simulink model "ModeAdjust"  (R2018b)
settings: Solver=FixedStepDiscrete  StartTime=0.0  StopTime=inf  FixedStep=0.01  RelTol=1e-3
undefined symbols (not defined in the file or in its folder): IfKeSMSbSeatMovBkRclnEnable_Val, IfKeSMSbSeatMovFrwdBkwdEnable_Val, IfKeSMSbSeatMovFtrstEnable_Val, IfKeSMSbSeatMovHdrstFrwdBkwdEnable_Val, IfKeSMSbSeatMovHdUpwdDnwdEnable_Val, IfKeSMSbSeatMovLgrstEnable_Val, IfKeSMSbSeatMovLtwdRtwdEnable_Val, IfVeSMSeStNumConfig, KeSMSbArmscreenMovEnable_Val, KeSMSbSeatMovLgrstExpdEnable_Val, KeSMSuFirstRwStBackPosDelta_Val, KeSMSuFirstRwStBackPosTolr_Val, KeSMSuFirstRwStCushFrntPosDelta_Val, KeSMSuFirstRwStCushFrntPosTolr_Val, KeSMSuFirstRwStCushRePosDelta_Val, KeSMSuFirstRwStCushRePosTolr_Val, KeSMSuFirstRwStFootrestPosDelta_Val, KeSMSuFirstRwStFootrestPosTolr_Val, KeSMSuFirstRwStFwdBkwdPosDelta_Val, KeSMSuFirstRwStFwdBkwdPosTolr_Val, KeSMSuMdMotFinshdTm_Val, KeSMSuMdRetryTm1_Val, KeSMSuModeReqDurgTm_Val, KeSMSuSecRwStArmTochPosDelta_Val, KeSMSuSecRwStArmTochPosTolr_Val, KeSMSuSecRwStBackPosDelta_Val, KeSMSuSecRwStBackPosTolr_Val, KeSMSuSecRwStFtrstUpwdDnwdPosDelta_Val, KeSMSuSecRwStFtrstUpwdDnwdPosTolr_Val, KeSMSuSecRwStFwdBkwdPosDelta_Val, KeSMSuSecRwStFwdBkwdPosTolr_Val, KeSMSuSecRwStHeadrestFwdBkwdPosDelta_Val, KeSMSuSecRwStHeadrestFwdBkwdPosTolr_Val, KeSMSuSecRwStHeadrestUpwdDwnwdPosDelta_Val, KeSMSuSecRwStHeadrestUpwdDwnwdPosTolr_Val, KeSMSuSecRwStLegrestInOutPosDelta_Val, KeSMSuSecRwStLegrestInOutPosTolr_Val, KeSMSuSecRwStLegrestUpwdDwnwdPosDelta_Val, KeSMSuSecRwStLegrestUpwdDwnwdPosTolr_Val, KeSMSuSecRwStLwdRwdPosDelta_Val, KeSMSuSecRwStLwdRwdPosTolr_Val, KeSMSuSecRwStVIPFtrstRefAngle_Val, KeSMSuThirdRwStFwdBkwdPosDelta_Val, KeSMSuThirdRwStFwdBkwdPosTolr_Val, KeSMSuThrdRwCushFoldPosDelta_Val, KeSMSuThrdRwCushFoldPosTolr_Val, KeSMSuThrdRwStBackPosDelta_Val, KeSMSuThrdRwStBackPosTolr_Val, KeSMSw4SLegrstCloseMdSecRwLtStFtrstUpwdDnwdPos_Val, KeSMSw4SLegrstCloseMdSecRwLtStFtrstUpwdDnwdPosMax_Val, KeSMSw4SLegrstCloseMdSecRwLtStFtrstUpwdDnwdPosMin_Val, KeSMSw4SLegrstCloseMdSecRwLtStLgrstOtwdInwdPos_Val, KeSMSw4SLegrstCloseMdSecRwLtStLgrstOtwdInwdPosMax_Val, KeSMSw4SLegrstCloseMdSecRwLtStLgrstOtwdInwdPosMin_Val, KeSMSw4SLegrstCloseMdSecRwLtStLgrstUpwdDnwdPos_Val, KeSMSw4SLegrstCloseMdSecRwLtStLgrstUpwdDnwdPosMax_Val, KeSMSw4SLegrstCloseMdSecRwLtStLgrstUpwdDnwdPosMin_Val, KeSMSw4SLegrstCloseMdSecRwRtStFtrstUpwdDnwdPos_Val, KeSMSw4SLegrstCloseMdSecRwRtStFtrstUpwdDnwdPosMax_Val, KeSMSw4SLegrstCloseMdSecRwRtStFtrstUpwdDnwdPosMin_Val ... (+1138)
libraries: Lib x401
(part 35 of 35)

== stateflow chart ModeAdjust/ModeAdjustRunnable_sys/ModeAdjust/RecvyR4s/Chart ==
  (default) -> (junction 3) : {failflg=0;}
  (junction 3) -> (junction 5) [order 1] : [!R2Lt_ini]
  (junction 5) -> (junction 9) [order 1] : [R2Lt_done]
  (junction 3) -> (junction 13) [order 2] : {R2Lt_En=false;}
  (junction 5) -> (junction 7) [order 2] : {R2Lt_En=true;}
  (junction 9) -> (junction 11) : {R2Lt_En=false;}
  (junction 7) -> (junction 13)
  (junction 11) -> (junction 7)
  (junction 13) -> (junction 237)
  (junction 237) -> (junction 244) [order 1] : [!HdUp_ini]
  (junction 244) -> (junction 234) [order 1] : [HdUp_Done]
  (junction 237) -> (junction 235) [order 2] : {HdUp_En =false;}
  (junction 244) -> (junction 246) [order 2] : {HdUp_En = true;}
  (junction 234) -> (junction 236) : {HdUp_En =false;}
  (junction 246) -> (junction 235)
  (junction 236) -> (junction 246)
  (junction 235) -> (junction 62)
  (junction 62) -> (junction 105) [order 1] : [!Step1_ini]
  (junction 105) -> (junction 107) [order 1] : [Step1done]
  (junction 62) -> (junction 68) [order 2] : {
      | StepEn_LgrstStep1=false;
      | }
  (junction 105) -> (junction 82) [order 2] : {StepEn_LgrstStep1=true;}
  (junction 107) -> (junction 109) : {StepEn_LgrstStep1=false;}
  (junction 82) -> (junction 68)
  (junction 109) -> (junction 82)
  (junction 68) -> (junction 143)
  (junction 143) -> (junction 142) [order 1] : [!Step2_ini]
  (junction 142) -> (junction 157) [order 1] : [downpos<=closedownpos2&&Ftpos>=FtposDelta]
  (junction 157) -> (junction 224) [order 1] : [Step1done&&Step3done]
  (junction 143) -> (junction 89) [order 2] : {
      | StepEn_LgrstStep2=false;
      | }
  (junction 142) -> (junction 154) [order 2]
  (junction 157) -> (junction 159) [order 2] : {
      | StepEn_LgrstStep2=false;
      | }
  (junction 224) -> (junction 228) : {failflg=1;}
  (junction 154) -> (junction 148) [order 1] : [downpos<closedownpos1&&Otpos>closeOtpos1]
  (junction 154) -> (junction 87) [order 2]
  (junction 148) -> (junction 150) : {StepEn_LgrstStep2 = false;}
  (junction 87) -> (junction 94) [order 1] : [Step2done]
  (junction 87) -> (junction 91) [order 2] : {
      | StepEn_LgrstStep2=true;
      | }
  (junction 94) -> (junction 96) : {
      | StepEn_LgrstStep2=false;
      | }
  (junction 91) -> (junction 89)
  (junction 96) -> (junction 91)
  (junction 150) -> (junction 96)
  (junction 159) -> (junction 150)
  (junction 228) -> (junction 159)
  (junction 89) -> (junction 101)
  (junction 101) -> (junction 113) [order 1] : [!Step3_ini]
  (junction 113) -> (junction 115) [order 1] : [Step3done||!Step1done]
  (junction 101) -> (junction 118) [order 2] : {
      | StepEn_LgrstStep3=false;
      | }
  (junction 113) -> (junction 258) [order 2]
  (junction 115) -> (junction 122) : {
      | StepEn_LgrstStep3=false;
      | }
  (junction 258) -> (junction 260) [order 1] : [downpos>closedownpos2]
  (junction 260) -> (junction 274) [order 1] : [Step2done]
  (junction 258) -> (junction 116) [order 2] : {
      | StepEn_LgrstStep3=true;
      | }
  (junction 260) -> (junction 262) [order 2] : {StepEn_LgrstStep3 = false;}
  (junction 274) -> (junction 276) : {
      | StepEn_LgrstStep3=true;
      | }
  (junction 116) -> (junction 118)
  (junction 262) -> (junction 116)
  (junction 276) -> (junction 262)
  (junction 122) -> (junction 276)
  (junction 118) -> (junction 182)
  (junction 182) -> (junction 178) [order 1] : [(Step1done&&Step2done&&Step3done)||failflg==1]
  (junction 178) -> (junction 252) [order 1] : [!HFwd_ini]
  (junction 252) -> (junction 173) [order 1] : [HdFwd_Done]
  (junction 182) -> (junction 181) [order 2]
  (junction 178) -> (junction 174) [order 2] : {HdFwd_En =false;}
  (junction 252) -> (junction 254) [order 2] : {HdFwd_En =true;}
  (junction 173) -> (junction 175) : {HdFwd_En =false;}
  (junction 254) -> (junction 174)
  (junction 175) -> (junction 254)
  (junction 174) -> (junction 176)
  (junction 176) -> (junction 181)
  (junction 181) -> (junction 165)
  data: R2Lt_ini input boolean; R2Lt_done input boolean; R2Lt_En output boolean; downpos input uint16; Otpos input uint16; Ftpos input uint16; closedownpos1 input uint16; closedownpos2 input uint16; closeOtpos1 input uint16; Step1done input boolean; Step2done input boolean; Step3done input boolean; Step1_ini input boolean; Step2_ini input boolean; Step3_ini input boolean; StepEn_LgrstStep1 output boolean; StepEn_LgrstStep2 output boolean; StepEn_LgrstStep3 output boolean; FtposDelta input uint16; HdFwd_Done input boolean; HdUp_Done input boolean; HdUp_En output boolean; HdFwd_En output boolean; OtposDelta input uint16; failflg output boolean; HdUp_ini input boolean; HFwd_ini input boolean

== stateflow chart ModeAdjust/ModeAdjustRunnable_sys/ModeAdjust/RecvyR4s/Chart1 ==
  (default) -> (junction 1)
  (junction 1) -> (junction 3) [order 1] : [Left_Done]
  (junction 1) -> (junction 7) [order 2] : {
      | IfVeSMSuSecRwLtStRclCmdSrv_Val_write=IfVeSMSuSecRwLtStRclCmdSrv_Val_writeRaw;
      | Md_L_DoneOk=false;
      | Md_L_DoneFailed=false;
      | }
  (junction 3) -> (junction 5) : {
      | IfVeSMSuSecRwLtStRclCmdSrv_Val_write=false;
      | Md_L_DoneOk=Md_L_DoneOkRaw;
      | Md_L_DoneFailed=Md_L_DoneFailedRaw;
      | }
  (junction 5) -> (junction 7)
  (junction 7) -> (junction 10)
  data: Left_Done input boolean; IfVeSMSuSecRwLtStRclCmdSrv_Val_write output boolean; IfVeSMSuSecRwLtStRclCmdSrv_Val_writeRaw input; Md_L_DoneOkRaw input; Md_L_DoneFailedRaw input; Md_L_DoneOk output boolean; Md_L_DoneFailed output boolean

== stateflow chart ModeAdjust/ModeAdjustRunnable_sys/ModeAdjust/INTMR/Chart ==
  (default) -> (junction 10)
  (junction 10) -> (junction 58) [order 1] : [!L_R2_ini]
  (junction 58) -> (junction 25) [order 1] : [L_R2_done]
  (junction 10) -> (junction 26) [order 2] : {L_R2_en=false;}
  (junction 58) -> (junction 35) [order 2] : {L_R2_en=true;}
  (junction 25) -> (junction 18) : {
      | L_R2_en=false;
      | }
  (junction 35) -> (junction 26)
  (junction 18) -> (junction 35)
  (junction 26) -> (junction 129)
  (junction 129) -> (junction 133) [order 1] : [!R_R2_ini]
  (junction 133) -> (junction 128) [order 1] : [R_R2_done]
  (junction 129) -> (junction 131) [order 2] : {R_R2_en=false;}
  (junction 133) -> (junction 127) [order 2] : {R_R2_en=true;}
  (junction 128) -> (junction 125) : {
      | R_R2_en=false;
      | }
  (junction 127) -> (junction 131)
  (junction 125) -> (junction 127)
  (junction 131) -> (junction 134)
  data: L_R2_ini input boolean; L_R2_done input boolean; R_R2_en output boolean; L_R2_en output boolean; R_R2_ini input boolean; R_R2_done input boolean

== stateflow chart ModeAdjust/ModeAdjustRunnable_sys/ModeAdjust/INTMR/Chart1 ==
  (default) -> (junction 1)
  (junction 1) -> (junction 3) [order 1] : [StepAlldone]
  (junction 1) -> (junction 7) [order 2] : {
      | IfVeSMSbSecRwRtStRclCmdSrv_Val_write=IfVeSMSbSecRwRtStRclCmdSrv_Val_writeRaw;
      | IfVeSMSuSecRwLtStRclCmdSrv_Val_write=IfVeSMSuSecRwLtStRclCmdSrv_Val_writeRaw;
      | isINTMDoneOk=false;
      | isINTMDoneFailed=false;
      | }
  (junction 3) -> (junction 5) : {
      | IfVeSMSbSecRwRtStRclCmdSrv_Val_write=false;
      | IfVeSMSuSecRwLtStRclCmdSrv_Val_write=false;
      | isINTMDoneOk=isINTMDoneOkRaw;
      | isINTMDoneFailed=isINTMDoneFailedRaw;
      | }
  (junction 5) -> (junction 7)
  (junction 7) -> (junction 10)
  data: StepAlldone input boolean; IfVeSMSbSecRwRtStRclCmdSrv_Val_write output boolean; IfVeSMSuSecRwLtStRclCmdSrv_Val_write output boolean; isINTMDoneOk output boolean; isINTMDoneFailed output boolean; IfVeSMSbSecRwRtStRclCmdSrv_Val_writeRaw input; IfVeSMSuSecRwLtStRclCmdSrv_Val_writeRaw input; isINTMDoneFailedRaw input; isINTMDoneOkRaw input

== stateflow chart ModeAdjust/ModeAdjustRunnable_sys/ModeAdjust/LgrstCloseL/Chart ==
  (default) -> (junction 62) : {failflg=0;}
  (junction 62) -> (junction 105) [order 1] : [!Step1_ini]
  (junction 105) -> (junction 107) [order 1] : [Step1done]
  (junction 62) -> (junction 68) [order 2] : {
      | StepEn_LgrstStep1=false;
      | }
  (junction 105) -> (junction 82) [order 2] : {StepEn_LgrstStep1=true;}
  (junction 107) -> (junction 109) : {StepEn_LgrstStep1=false;}
  (junction 82) -> (junction 68)
  (junction 109) -> (junction 82)
  (junction 68) -> (junction 143)
  (junction 143) -> (junction 142) [order 1] : [!Step2_ini]
  (junction 142) -> (junction 157) [order 1] : [downpos<=closedownpos2&&Ftpos>=FtposDelta]
  (junction 157) -> (junction 224) [order 1] : [Step1done&&Step3done]
  (junction 143) -> (junction 89) [order 2] : {
      | StepEn_LgrstStep2=false;
      | }
  (junction 142) -> (junction 154) [order 2]
  (junction 157) -> (junction 159) [order 2] : {
      | StepEn_LgrstStep2=false;
      | }
  (junction 224) -> (junction 228) : {failflg=1;}
  (junction 154) -> (junction 148) [order 1] : [downpos<closedownpos1&&Otpos>closeOtpos1]
  (junction 154) -> (junction 87) [order 2]
  (junction 148) -> (junction 150) : {StepEn_LgrstStep2 = false;}
  (junction 87) -> (junction 94) [order 1] : [Step2done]
  (junction 87) -> (junction 91) [order 2] : {
      | StepEn_LgrstStep2=true;
      | }
  (junction 94) -> (junction 96) : {
      | StepEn_LgrstStep2=false;
      | }
  (junction 91) -> (junction 89)
  (junction 96) -> (junction 91)
  (junction 150) -> (junction 96)
  (junction 159) -> (junction 150)
  (junction 228) -> (junction 159)
  (junction 89) -> (junction 101)
  (junction 101) -> (junction 113) [order 1] : [!Step3_ini]
  (junction 113) -> (junction 115) [order 1] : [Step3done||!Step1done]
  (junction 101) -> (junction 118) [order 2] : {
      | StepEn_LgrstStep3=false;
      | }
  (junction 113) -> (junction 215) [order 2]
  (junction 115) -> (junction 122) : {
      | StepEn_LgrstStep3=false;
      | }
  (junction 215) -> (junction 217) [order 1] : [downpos>closedownpos2]
  (junction 217) -> (junction 259) [order 1] : [Step2done]
  (junction 215) -> (junction 116) [order 2] : {
      | StepEn_LgrstStep3=true;
      | }
  (junction 217) -> (junction 219) [order 2] : {
      | StepEn_LgrstStep3=false;
      | }
  (junction 259) -> (junction 261) : {
      | StepEn_LgrstStep3=true;
      | }
  (junction 116) -> (junction 118)
  (junction 219) -> (junction 116)
  (junction 261) -> (junction 219)
  (junction 122) -> (junction 261)
  (junction 118) -> (junction 182)
  data: downpos input uint16; Otpos input uint16; Ftpos input uint16; closedownpos1 input uint16; closedownpos2 input uint16; closeOtpos1 input uint16; Step1done input boolean; Step2done input boolean; Step3done input boolean; Step1_ini input boolean; Step2_ini input boolean; Step3_ini input boolean; StepEn_LgrstStep1 output boolean; StepEn_LgrstStep2 output boolean; StepEn_LgrstStep3 output boolean; FtposDelta input uint16; OtposDelta input uint16; failflg output boolean

== stateflow chart ModeAdjust/ModeAdjustRunnable_sys/ModeAdjust/LgrstCloseL/Chart1 ==
  (default) -> (junction 1)
  (junction 1) -> (junction 3) [order 1] : [Left_Done]
  (junction 1) -> (junction 7) [order 2] : {
      | IfVeSMSuSecRwLtStRclCmdSrv_Val_write=IfVeSMSuSecRwLtStRclCmdSrv_Val_writeRaw;
      | Md_L_DoneOk=false;
      | Md_L_DoneFailed=false;
      | }
  (junction 3) -> (junction 5) : {
      | IfVeSMSuSecRwLtStRclCmdSrv_Val_write=false;
      | Md_L_DoneOk=Md_L_DoneOkRaw;
      | Md_L_DoneFailed=Md_L_DoneFailedRaw;
      | }
  (junction 5) -> (junction 7)
  (junction 7) -> (junction 10)
  data: Left_Done input boolean; IfVeSMSuSecRwLtStRclCmdSrv_Val_write output boolean; IfVeSMSuSecRwLtStRclCmdSrv_Val_writeRaw input; Md_L_DoneOkRaw input; Md_L_DoneFailedRaw input; Md_L_DoneOk output boolean; Md_L_DoneFailed output boolean

== stateflow chart ModeAdjust/ModeAdjustRunnable_sys/ModeAdjust/LgrstOpenL/Chart ==
  (default) -> (junction 182) : {failflg =0;}
  (junction 182) -> (junction 62)
  (junction 62) -> (junction 76) [order 1] : [!Step1_ini]
  (junction 76) -> (junction 64) [order 1] : [pos<openpos1]
  (junction 64) -> (junction 74) [order 1] : [Step1done]
  (junction 62) -> (junction 68) [order 2] : {
      | StepEn_LgrstStep1=false;
      | }
  (junction 76) -> (junction 105) [order 2]
  (junction 64) -> (junction 66) [order 2] : {
      | StepEn_LgrstStep1=true;
      | StepEn_LgrstStep2=false;
      | StepEn_LgrstStep3=false;
      | }
  (junction 74) -> (junction 102) : {
      | StepEn_LgrstStep1=false;
      | StepEn_LgrstStep2=false;
      | StepEn_LgrstStep3=false;
      | failflg =1;
      | }
  (junction 105) -> (junction 107) [order 1] : [!Step2done||Step1done]
  (junction 105) -> (junction 82) [order 2] : {StepEn_LgrstStep1=true;}
  (junction 107) -> (junction 109) : {StepEn_LgrstStep1=false;}
  (junction 82) -> (junction 68)
  (junction 109) -> (junction 82)
  (junction 102) -> (junction 66)
  (junction 68) -> (junction 85)
  (junction 66) -> (junction 99)
  (junction 85) -> (junction 87) [order 1] : [!Step2_ini]
  (junction 87) -> (junction 94) [order 1] : [Step2done]
  (junction 85) -> (junction 89) [order 2] : {
      | StepEn_LgrstStep2=false;
      | }
  (junction 87) -> (junction 91) [order 2] : {
      | StepEn_LgrstStep2=true;
      | }
  (junction 94) -> (junction 96) : {
      | StepEn_LgrstStep2=false;
      | }
  (junction 91) -> (junction 89)
  (junction 96) -> (junction 91)
  (junction 89) -> (junction 101)
  (junction 101) -> (junction 113) [order 1] : [!Step3_ini]
  (junction 113) -> (junction 115) [order 1] : [(!Step2done)||Step3done]
  (junction 101) -> (junction 118) [order 2] : {
      | StepEn_LgrstStep3=false;
      | }
  (junction 113) -> (junction 116) [order 2] : {
      | StepEn_LgrstStep3=true;
      | }
  (junction 115) -> (junction 122) : {
      | StepEn_LgrstStep3=false;
      | }
  (junction 116) -> (junction 118)
  (junction 122) -> (junction 116)
  (junction 99) -> (junction 122)
  (junction 118) -> (junction 166)
  data: pos input uint16; openpos1 input uint16; Step1done input boolean; Step2done input boolean; Step3done input boolean; Step1_ini input boolean; Step2_ini input boolean; Step3_ini input boolean; StepEn_LgrstStep1 output boolean; StepEn_LgrstStep2 output boolean; StepEn_LgrstStep3 output boolean; failflg output boolean

== stateflow chart ModeAdjust/ModeAdjustRunnable_sys/ModeAdjust/LgrstOpenL/Chart1 ==
  (default) -> (junction 1)
  (junction 1) -> (junction 3) [order 1] : [Left_Done]
  (junction 1) -> (junction 7) [order 2] : {
      | IfVeSMSuSecRwLtStRclCmdSrv_Val_write=IfVeSMSuSecRwLtStRclCmdSrv_Val_writeRaw;
      | Md_L_DoneOk=false;
      | Md_L_DoneFailed=false;
      | }
  (junction 3) -> (junction 5) : {
      | IfVeSMSuSecRwLtStRclCmdSrv_Val_write=false;
      | Md_L_DoneOk=Md_L_DoneOkRaw;
      | Md_L_DoneFailed=Md_L_DoneFailedRaw;
      | }
  (junction 5) -> (junction 7)
  (junction 7) -> (junction 10)
  data: Left_Done input boolean; IfVeSMSuSecRwLtStRclCmdSrv_Val_write output boolean; IfVeSMSuSecRwLtStRclCmdSrv_Val_writeRaw input; Md_L_DoneOkRaw input; Md_L_DoneFailedRaw input; Md_L_DoneOk output boolean; Md_L_DoneFailed output boolean

== stateflow chart ModeAdjust/ModeAdjustRunnable_sys/ModeAdjust/LgrstOpenR/Chart ==
  (default) -> (junction 182) : {failflg =0;}
  (junction 182) -> (junction 62)
  (junction 62) -> (junction 76) [order 1] : [!Step1_ini]
  (junction 76) -> (junction 64) [order 1] : [pos<openpos1]
  (junction 64) -> (junction 74) [order 1] : [Step1done]
  (junction 62) -> (junction 68) [order 2] : {
      | StepEn_LgrstStep1=false;
      | }
  (junction 76) -> (junction 105) [order 2]
  (junction 64) -> (junction 66) [order 2] : {
      | StepEn_LgrstStep1=true;
      | StepEn_LgrstStep2=false;
      | StepEn_LgrstStep3=false;
      | }
  (junction 74) -> (junction 102) : {
      | StepEn_LgrstStep1=false;
      | StepEn_LgrstStep2=false;
      | StepEn_LgrstStep3=false;
      | failflg =1;
      | }
  (junction 105) -> (junction 107) [order 1] : [!Step2done||Step1done]
  (junction 105) -> (junction 82) [order 2] : {StepEn_LgrstStep1=true;}
  (junction 107) -> (junction 109) : {StepEn_LgrstStep1=false;}
  (junction 82) -> (junction 68)
  (junction 109) -> (junction 82)
  (junction 102) -> (junction 66)
  (junction 68) -> (junction 85)
  (junction 66) -> (junction 99)
  (junction 85) -> (junction 87) [order 1] : [!Step2_ini]
  (junction 87) -> (junction 94) [order 1] : [Step2done]
  (junction 85) -> (junction 89) [order 2] : {
      | StepEn_LgrstStep2=false;
      | }
  (junction 87) -> (junction 91) [order 2] : {
      | StepEn_LgrstStep2=true;
      | }
  (junction 94) -> (junction 96) : {
      | StepEn_LgrstStep2=false;
      | }
  (junction 91) -> (junction 89)
  (junction 96) -> (junction 91)
  (junction 89) -> (junction 101)
  (junction 101) -> (junction 113) [order 1] : [!Step3_ini]
  (junction 113) -> (junction 115) [order 1] : [(!Step2done)||Step3done]
  (junction 101) -> (junction 118) [order 2] : {
      | StepEn_LgrstStep3=false;
      | }
  (junction 113) -> (junction 116) [order 2] : {
      | StepEn_LgrstStep3=true;
      | }
  (junction 115) -> (junction 122) : {
      | StepEn_LgrstStep3=false;
      | }
  (junction 116) -> (junction 118)
  (junction 122) -> (junction 116)
  (junction 99) -> (junction 122)
  (junction 118) -> (junction 166)
  data: pos input uint16; openpos1 input uint16; Step1done input boolean; Step2done input boolean; Step3done input boolean; Step1_ini input boolean; Step2_ini input boolean; Step3_ini input boolean; StepEn_LgrstStep1 output boolean; StepEn_LgrstStep2 output boolean; StepEn_LgrstStep3 output boolean; failflg output boolean

== stateflow chart ModeAdjust/ModeAdjustRunnable_sys/ModeAdjust/LgrstOpenR/Chart1 ==
  (default) -> (junction 1)
  (junction 1) -> (junction 3) [order 1] : [Left_Done]
  (junction 1) -> (junction 7) [order 2] : {
      | IfVeSMSuSecRwLtStRclCmdSrv_Val_write=IfVeSMSuSecRwLtStRclCmdSrv_Val_writeRaw;
      | Md_L_DoneOk=false;
      | Md_L_DoneFailed=false;
      | }
  (junction 3) -> (junction 5) : {
      | IfVeSMSuSecRwLtStRclCmdSrv_Val_write=false;
      | Md_L_DoneOk=Md_L_DoneOkRaw;
      | Md_L_DoneFailed=Md_L_DoneFailedRaw;
      | }
  (junction 5) -> (junction 7)
  (junction 7) -> (junction 10)
  data: Left_Done input boolean; IfVeSMSuSecRwLtStRclCmdSrv_Val_write output boolean; IfVeSMSuSecRwLtStRclCmdSrv_Val_writeRaw input; Md_L_DoneOkRaw input; Md_L_DoneFailedRaw input; Md_L_DoneOk output boolean; Md_L_DoneFailed output boolean

== stateflow chart ModeAdjust/ModeAdjustRunnable_sys/ModeAdjust/LgrstCloseR/Chart ==
  (default) -> (junction 62) : {failflg=0;}
  (junction 62) -> (junction 105) [order 1] : [!Step1_ini]
  (junction 105) -> (junction 107) [order 1] : [Step1done]
  (junction 62) -> (junction 68) [order 2] : {
      | StepEn_LgrstStep1=false;
      | }
  (junction 105) -> (junction 82) [order 2] : {StepEn_LgrstStep1=true;}
  (junction 107) -> (junction 109) : {StepEn_LgrstStep1=false;}
  (junction 82) -> (junction 68)
  (junction 109) -> (junction 82)
  (junction 68) -> (junction 143)
  (junction 143) -> (junction 142) [order 1] : [!Step2_ini]
  (junction 142) -> (junction 157) [order 1] : [downpos<=closedownpos2&&Ftpos>=FtposDelta]
  (junction 157) -> (junction 224) [order 1] : [Step1done&&Step3done]
  (junction 143) -> (junction 89) [order 2] : {
      | StepEn_LgrstStep2=false;
      | }
  (junction 142) -> (junction 154) [order 2]
  (junction 157) -> (junction 159) [order 2] : {
      | StepEn_LgrstStep2=false;
      | }
  (junction 224) -> (junction 228) : {failflg=1;}
  (junction 154) -> (junction 148) [order 1] : [downpos<closedownpos1&&Otpos>closeOtpos1]
  (junction 154) -> (junction 87) [order 2]
  (junction 148) -> (junction 150) : {StepEn_LgrstStep2 = false;}
  (junction 87) -> (junction 94) [order 1] : [Step2done]
  (junction 87) -> (junction 91) [order 2] : {
      | StepEn_LgrstStep2=true;
      | }
  (junction 94) -> (junction 96) : {
      | StepEn_LgrstStep2=false;
      | }
  (junction 91) -> (junction 89)
  (junction 96) -> (junction 91)
  (junction 150) -> (junction 96)
  (junction 159) -> (junction 150)
  (junction 228) -> (junction 159)
  (junction 89) -> (junction 101)
  (junction 101) -> (junction 113) [order 1] : [!Step3_ini]
  (junction 113) -> (junction 115) [order 1] : [Step3done||!Step1done]
  (junction 101) -> (junction 118) [order 2] : {
      | StepEn_LgrstStep3=false;
      | }
  (junction 113) -> (junction 215) [order 2]
  (junction 115) -> (junction 122) : {
      | StepEn_LgrstStep3=false;
      | }
  (junction 215) -> (junction 217) [order 1] : [downpos>closedownpos2]
  (junction 217) -> (junction 259) [order 1] : [Step2done]
  (junction 215) -> (junction 116) [order 2] : {
      | StepEn_LgrstStep3=true;
      | }
  (junction 217) -> (junction 219) [order 2] : {
      | StepEn_LgrstStep3=false;
      | }
  (junction 259) -> (junction 261) : {
      | StepEn_LgrstStep3=true;
      | }
  (junction 116) -> (junction 118)
  (junction 219) -> (junction 116)
  (junction 261) -> (junction 219)
  (junction 122) -> (junction 261)
  (junction 118) -> (junction 182)
  data: downpos input uint16; Otpos input uint16; Ftpos input uint16; closedownpos1 input uint16; closedownpos2 input uint16; closeOtpos1 input uint16; Step1done input boolean; Step2done input boolean; Step3done input boolean; Step1_ini input boolean; Step2_ini input boolean; Step3_ini input boolean; StepEn_LgrstStep1 output boolean; StepEn_LgrstStep2 output boolean; StepEn_LgrstStep3 output boolean; FtposDelta input uint16; OtposDelta input uint16; failflg output boolean

== stateflow chart ModeAdjust/ModeAdjustRunnable_sys/ModeAdjust/LgrstCloseR/Chart1 ==
  (default) -> (junction 1)
  (junction 1) -> (junction 3) [order 1] : [Left_Done]
  (junction 1) -> (junction 7) [order 2] : {
      | IfVeSMSuSecRwLtStRclCmdSrv_Val_write=IfVeSMSuSecRwLtStRclCmdSrv_Val_writeRaw;
      | Md_L_DoneOk=false;
      | Md_L_DoneFailed=false;
      | }
  (junction 3) -> (junction 5) : {
      | IfVeSMSuSecRwLtStRclCmdSrv_Val_write=false;
      | Md_L_DoneOk=Md_L_DoneOkRaw;
      | Md_L_DoneFailed=Md_L_DoneFailedRaw;
      | }
  (junction 5) -> (junction 7)
  (junction 7) -> (junction 10)
  data: Left_Done input boolean; IfVeSMSuSecRwLtStRclCmdSrv_Val_write output boolean; IfVeSMSuSecRwLtStRclCmdSrv_Val_writeRaw input; Md_L_DoneOkRaw input; Md_L_DoneFailedRaw input; Md_L_DoneOk output boolean; Md_L_DoneFailed output boolean

== stateflow chart ModeAdjust/ModeAdjustRunnable_sys/ModeAdjust/AcsMdEntry/Chart1 ==
  (default) -> (junction 1)
  (junction 1) -> (junction 3) [order 1] : [StepAlldone]
  (junction 1) -> (junction 25) [order 2] : {
      | IfVeSMSbSecRwRtStRclCmdSrv_Val_write=true;
      | IfVeSMSuSecRwLtStRclCmdSrv_Val_write=true;
      | IfVeSMSbDrvStRclCmdSrv_Val_write=true;
      | IfVeSMSuPassStRclCmdSrv_Val_write=true;
      | isAcsMdEntryDoneOk=false;
      | isAcsMdEntryDoneFailed=false;
      | }
  (junction 3) -> (junction 5) : {
      | IfVeSMSbThdRwRtStRclCmdSrv_Val_write=false;
      | IfVeSMSbThdRwLtStRclCmdSrv_Val_write=false;
      | IfVeSMSbSecRwRtStRclCmdSrv_Val_write=false;
      | IfVeSMSuSecRwLtStRclCmdSrv_Val_write=false;
      | IfVeSMSbDrvStRclCmdSrv_Val_write=false;
      | IfVeSMSuPassStRclCmdSrv_Val_write=false;
      | isAcsMdEntryDoneOk=isAcsMdEntryDoneOkRaw;
      | isAcsMdEntryDoneFailed=isAcsMdEntryDoneFailedRaw;
      | }
  (junction 25) -> (junction 26) [order 1] : [isRightSeatOccupied]
  (junction 25) -> (junction 30) [order 2] : {IfVeSMSbThdRwRtStRclCmdSrv_Val_write=true;}
  (junction 26) -> (junction 28) : {IfVeSMSbThdRwRtStRclCmdSrv_Val_write=false;}
  (junction 28) -> (junction 30)
  (junction 30) -> (junction 33)
  (junction 33) -> (junction 35) [order 1] : [isLeftSeatOccupied]
  (junction 33) -> (junction 41) [order 2] : {IfVeSMSbThdRwLtStRclCmdSrv_Val_write=true;}
  (junction 35) -> (junction 39) : {IfVeSMSbThdRwLtStRclCmdSrv_Val_write=false;}
  (junction 39) -> (junction 41)
  (junction 41) -> (junction 7)
  (junction 5) -> (junction 7)
  (junction 7) -> (junction 10)
  data: StepAlldone input boolean; IfVeSMSbThdRwRtStRclCmdSrv_Val_write output boolean; IfVeSMSbThdRwLtStRclCmdSrv_Val_write output boolean; IfVeSMSbSecRwRtStRclCmdSrv_Val_write output boolean; IfVeSMSuSecRwLtStRclCmdSrv_Val_write output boolean; IfVeSMSbDrvStRclCmdSrv_Val_write output boolean; IfVeSMSuPassStRclCmdSrv_Val_write output boolean; IfVeSMSbThdRwRtStRclCmdSrv_Val_writeRaw input; IfVeSMSbThdRwLtStRclCmdSrv_Val_writeRaw input; isAcsMdEntryDoneOk output boolean; isAcsMdEntryDoneFailed output boolean; isAcsMdEntryDoneFailedRaw input; isAcsMdEntryDoneOkRaw input; isRightSeatOccupied input; isLeftSeatOccupied input

== stateflow chart ModeAdjust/ModeAdjustRunnable_sys/ModeAdjust/AcsMdExt/Chart ==
  (default) -> (junction 10)
  (junction 10) -> (junction 58) [order 1] : [!Stg1ini]
  (junction 58) -> (junction 25) [order 1] : [Stg1done]
  (junction 10) -> (junction 26) [order 2] : {Stg1Req=false;}
  (junction 58) -> (junction 35) [order 2] : {Stg1Req=true;}
  (junction 25) -> (junction 18) : {
      | Stg1Req=false;
      | }
  (junction 35) -> (junction 26)
  (junction 18) -> (junction 35)
  (junction 26) -> (junction 36)
  (junction 36) -> (junction 44) [order 1] : [!Stg2ini]
  (junction 44) -> (junction 33) [order 1] : [Stg2done]
  (junction 36) -> (junction 27) [order 2] : {
      | Stg2Req=false;
      | }
  (junction 44) -> (junction 45) [order 2] : {
      | Stg2Req=true;
      | }
  (junction 33) -> (junction 73) : {
      | Stg2Req=false;
      | }
  (junction 45) -> (junction 27)
  (junction 73) -> (junction 45)
  (junction 27) -> (junction 52)
  (junction 52) -> (junction 31)
  (junction 31) -> (junction 34) [order 1] : [Stg1Req==true]
  (junction 31) -> (junction 38) [order 2]
  (junction 34) -> (junction 47) : {
      | R2ST_right_Step1=true;
      | R2ST_left_Step1=true;
      | DrvST_Step1=true;
      | PassST_Step1=true;
      |
      | R2ST_right_Step2=false;
      | R2ST_left_Step2=false;
      | DrvST_Step2=false;
      | PassST_Step2=false;
      | }
  (junction 38) -> (junction 24) [order 1] : [Stg2Req==true]
  (junction 38) -> (junction 43) [order 2]
  (junction 24) -> (junction 72) : {
      | R2ST_right_Step1=false;
      | R2ST_left_Step1=false;
      | DrvST_Step1=false;
      | PassST_Step1=false;
      |
      | R2ST_right_Step2=true;
      | R2ST_left_Step2=true;
      | DrvST_Step2=true;
      | PassST_Step2=true;
      | }
  (junction 43) -> (junction 71) : {
      | R2ST_right_Step1=false;
      | R2ST_left_Step1=false;
      | DrvST_Step1=false;
      | PassST_Step1=false;
      |
      | R2ST_right_Step2=false;
      | R2ST_left_Step2=false;
      | DrvST_Step2=false;
      | PassST_Step2=false;
      | }
  (junction 61) -> (junction 71)
  (junction 72) -> (junction 61)
  (junction 47) -> (junction 72)
  (junction 71) -> (junction 48)
  data: Stg1ini input boolean; Stg2ini input boolean; Stg1done input boolean; Stg2done input boolean; Stg1Req output boolean; Stg2Req output boolean; R2ST_right_Step1 output boolean; R2ST_left_Step1 output boolean; DrvST_Step1 output boolean; PassST_Step1 output boolean; R2ST_right_Step2 output boolean; R2ST_left_Step2 output boolean; DrvST_Step2 output boolean; PassST_Step2 output boolean

== stateflow chart ModeAdjust/ModeAdjustRunnable_sys/ModeAdjust/AcsMdExt/Chart1 ==
  (default) -> (junction 1)
  (junction 1) -> (junction 3) [order 1] : [StepAlldone]
  (junction 1) -> (junction 7) [order 2] : {
      | IfVeSMSbSecRwRtStRclCmdSrv_Val_write=IfVeSMSbSecRwRtStRclCmdSrv_Val_writeRaw;
      | IfVeSMSuSecRwLtStRclCmdSrv_Val_write=IfVeSMSuSecRwLtStRclCmdSrv_Val_writeRaw;
      | IfVeSMSbDrvStRclCmdSrv_Val_write=IfVeSMSbDrvStRclCmdSrv_Val_writeRaw;
      | IfVeSMSuPassStRclCmdSrv_Val_write=IfVeSMSuPassStRclCmdSrv_Val_writeRaw;
      | isAcsMdEntryDoneOk=false;
      | isAcsMdEntryDoneFailed=false;
      | }
  (junction 3) -> (junction 5) : {
      | IfVeSMSbSecRwRtStRclCmdSrv_Val_write=false;
      | IfVeSMSuSecRwLtStRclCmdSrv_Val_write=false;
      | IfVeSMSbDrvStRclCmdSrv_Val_write=false;
      | IfVeSMSuPassStRclCmdSrv_Val_write=false;
      | isAcsMdEntryDoneOk=isAcsMdEntryDoneOkRaw;
      | isAcsMdEntryDoneFailed=isAcsMdEntryDoneFailedRaw;
      | }
  (junction 5) -> (junction 7)
  (junction 7) -> (junction 10)
  data: StepAlldone input boolean; IfVeSMSbSecRwRtStRclCmdSrv_Val_write output boolean; IfVeSMSuSecRwLtStRclCmdSrv_Val_write output boolean; IfVeSMSbDrvStRclCmdSrv_Val_write output boolean; IfVeSMSuPassStRclCmdSrv_Val_write output boolean; isAcsMdEntryDoneOk output boolean; isAcsMdEntryDoneFailed output boolean; IfVeSMSbSecRwRtStRclCmdSrv_Val_writeRaw input; IfVeSMSuSecRwLtStRclCmdSrv_Val_writeRaw input; IfVeSMSbDrvStRclCmdSrv_Val_writeRaw input; IfVeSMSuPassStRclCmdSrv_Val_writeRaw input; isAcsMdEntryDoneFailedRaw input; isAcsMdEntryDoneOkRaw input

== stateflow chart ModeAdjust/ModeAdjustRunnable_sys/ModeAdjust/VIPL/Chart2 ==
  (default) -> (junction 450)
  (junction 450) -> (junction 448) [order 1] : [!L_R3Step1_ini]
  (junction 448) -> (junction 454) [order 1] : [L_R3Step1done]
  (junction 450) -> (junction 451) [order 2] : {L_R3Step1=false;}
  (junction 448) -> (junction 453) [order 2] : {L_R3Step1=true;}
  (junction 454) -> (junction 449) : {L_R3Step1=false;}
  (junction 453) -> (junction 451)
  (junction 449) -> (junction 453)
  (junction 451) -> (junction 441)
  (junction 441) -> (junction 444) [order 1] : [!L_R2Step1_ini&&L_PosOvrup]
  (junction 444) -> (junction 443) [order 1] : [L_R2Step1done]
  (junction 441) -> (junction 445) [order 2] : {L_R2Step1=false;}
  (junction 444) -> (junction 446) [order 2] : {L_R2Step1=true;}
  (junction 443) -> (junction 467) : {L_R2Step1=false;}
  (junction 446) -> (junction 445)
  (junction 467) -> (junction 446)
  (junction 445) -> (junction 460)
  (junction 460) -> (junction 455) [order 1] : [!L_R2Step2_ini&&L_R2Step1done]
  (junction 455) -> (junction 465) [order 1] : [L_R2Step2done]
  (junction 460) -> (junction 463) [order 2] : {L_R2Step2=false;}
  (junction 455) -> (junction 459) [order 2] : {L_R2Step2=true;}
  (junction 465) -> (junction 464) : {L_R2Step2=false;}
  (junction 459) -> (junction 463)
  (junction 464) -> (junction 459)
  (junction 463) -> (junction 577)
  (junction 577) -> (junction 581) [order 1] : [!L_R1Step1_ini&&Stage1_done]
  (junction 581) -> (junction 582) [order 1] : [Stage2_done]
  (junction 577) -> (junction 578) [order 2] : {L_R1Step1=false;}
  (junction 581) -> (junction 580) [order 2] : {L_R1Step1=true;}
  (junction 582) -> (junction 579) : {L_R1Step1=false;}
  (junction 580) -> (junction 578)
  (junction 579) -> (junction 580)
  (junction 578) -> (junction 466)
  (junction 466) -> (junction 456) [order 1] : [!L_R2Step3_ini&&Stage1_done&&Stage2_done]
  (junction 456) -> (junction 461) [order 1] : [Stage3_done]
  (junction 466) -> (junction 462) [order 2] : {L_R2Step3=false;}
  (junction 456) -> (junction 457) [order 2] : {L_R2Step3=true;}
  (junction 461) -> (junction 458) : {L_R2Step3=false;}
  (junction 457) -> (junction 462)
  (junction 458) -> (junction 457)
  (junction 462) -> (junction 473)
  data: L_R3Step1 output boolean; L_R2Step1 output boolean; L_R2Step2 output boolean; L_R2Step3 output boolean; L_R3Step1_ini input boolean; L_R2Step1_ini input boolean; L_R2Step2_ini input boolean; L_R2Step3_ini input boolean; L_PosOvrup input boolean; L_R3Step1done input boolean; L_R2Step1done input boolean; L_R2Step2done input boolean; Stage1_done input boolean; Stage2_done input boolean; L_R1Step1_ini input boolean; L_R1Step1 output boolean; Stage3_done input boolean

== stateflow chart ModeAdjust/ModeAdjustRunnable_sys/ModeAdjust/VIPL/Chart1 ==
  (default) -> (junction 51)
  (junction 51) -> (junction 53) [order 1] : [LeftDone]
  (junction 51) -> (junction 7) [order 2] : {
      | IfVeSMSbThdRwLtStRclCmdSrv_Val_write=IfVeSMSbThdRwLtStRclCmdSrv_Val_writeRaw;
      | IfVeSMSuSecRwLtStRclCmdSrv_Val_write=IfVeSMSuSecRwLtStRclCmdSrv_Val_writeRaw;
      | IfVeSMSuDrvStRclCmdSrv_Val_write =IfVeSMSuDrvStRclCmdSrv_Val_writeRaw;
      | Md_L_DoneOk=false;
      | Md_L_DoneFailed=false;
      | }
  (junction 53) -> (junction 55) : {
      | IfVeSMSbThdRwLtStRclCmdSrv_Val_write=false;
      | IfVeSMSuSecRwLtStRclCmdSrv_Val_write=false;
      | IfVeSMSuDrvStRclCmdSrv_Val_write=false;
      | Md_L_DoneOk=Md_L_DoneOkRaw;
      | Md_L_DoneFailed=Md_L_DoneFailedRaw;
      | }
  (junction 55) -> (junction 7)
  (junction 7) -> (junction 46)
  data: LeftDone input boolean; IfVeSMSbThdRwLtStRclCmdSrv_Val_write output boolean; IfVeSMSuSecRwLtStRclCmdSrv_Val_write output boolean; IfVeSMSbThdRwLtStRclCmdSrv_Val_writeRaw input; IfVeSMSuSecRwLtStRclCmdSrv_Val_writeRaw input; Md_L_DoneOkRaw input; Md_L_DoneFailedRaw input; Md_L_DoneOk output boolean; Md_L_DoneFailed output boolean; IfVeSMSuDrvStRclCmdSrv_Val_writeRaw input; IfVeSMSuDrvStRclCmdSrv_Val_write output boolean

== stateflow chart ModeAdjust/ModeAdjustRunnable_sys/ModeAdjust/RecoveryL/Chart1 ==
  (default) -> (junction 1)
  (junction 1) -> (junction 3) [order 1] : [Left_Done]
  (junction 1) -> (junction 7) [order 2] : {
      | IfVeSMSuSecRwLtStRclCmdSrv_Val_write=IfVeSMSuSecRwLtStRclCmdSrv_Val_writeRaw;
      | IfVeSMSbDrvStRclCmdSrv_Val_write=true;
      | Md_L_DoneOk=false;
      | Md_L_DoneFailed=false;
      | }
  (junction 3) -> (junction 5) : {
      | IfVeSMSuSecRwLtStRclCmdSrv_Val_write=false;
      | IfVeSMSbDrvStRclCmdSrv_Val_write=false;
      | Md_L_DoneOk=Md_L_DoneOkRaw;
      | Md_L_DoneFailed=Md_L_DoneFailedRaw;
      | }
  (junction 5) -> (junction 7)
  (junction 7) -> (junction 10)
  data: Left_Done input boolean; IfVeSMSuSecRwLtStRclCmdSrv_Val_write output boolean; IfVeSMSuSecRwLtStRclCmdSrv_Val_writeRaw input boolean; Md_L_DoneOkRaw input boolean; Md_L_DoneFailedRaw input boolean; Md_L_DoneOk output boolean; Md_L_DoneFailed output boolean; IfVeSMSbDrvStRclCmdSrv_Val_write output boolean

== stateflow chart ModeAdjust/ModeAdjustRunnable_sys/ModeAdjust/RecoveryL/Chart ==
  (default) -> (junction 3)
  (junction 3) -> (junction 5) [order 1] : [!R2Lt_ini]
  (junction 5) -> (junction 9) [order 1] : [R2Lt_done]
  (junction 3) -> (junction 13) [order 2] : {R2Lt_En=false;}
  (junction 5) -> (junction 7) [order 2] : {R2Lt_En=true;}
  (junction 9) -> (junction 11) : {R2Lt_En=false;}
  (junction 7) -> (junction 13)
  (junction 11) -> (junction 7)
  (junction 13) -> (junction 65)
  (junction 65) -> (junction 66) [order 1] : [!Drv_ini]
  (junction 66) -> (junction 75) [order 1] : [Drv_done]
  (junction 65) -> (junction 72) [order 2] : {Drv_En=false;}
  (junction 66) -> (junction 70) [order 2] : {Drv_En=true;}
  (junction 75) -> (junction 71) : {Drv_En=false;}
  (junction 70) -> (junction 72)
  (junction 71) -> (junction 70)
  data: R2Lt_ini input boolean; R2Lt_done input boolean; R2Lt_En output boolean; Drv_ini input boolean; Drv_done input boolean; Drv_En output boolean

== stateflow chart ModeAdjust/ModeAdjustRunnable_sys/ModeAdjust/LugL/Chart ==
  (default) -> (junction 5)
  (junction 5) -> (junction 9) [order 1] : [!R3Lt_Step1_ini]
  (junction 9) -> (junction 49) [order 1] : [R3Lt_Step1_done]
  (junction 5) -> (junction 56) [order 2] : {R3Lt_Step1En=false;}
  (junction 9) -> (junction 53) [order 2] : {R3Lt_Step1En=true;}
  (junction 49) -> (junction 51) : {R3Lt_Step1En=false;}
  (junction 53) -> (junction 56)
  (junction 51) -> (junction 53)
  (junction 56) -> (junction 58)
  (junction 58) -> (junction 60) [order 1] : [(!R3Lt_Step2_ini)&&(R3Lt_Step1_done)]
  (junction 60) -> (junction 62) [order 1] : [R3Lt_Step2_done]
  (junction 58) -> (junction 7) [order 2] : {R3Lt_Step2En=false;}
  (junction 60) -> (junction 66) [order 2] : {R3Lt_Step2En=true;}
  (junction 62) -> (junction 64) : {R3Lt_Step2En=false;}
  (junction 66) -> (junction 7)
  (junction 64) -> (junction 66)
  data: R3Lt_Step1_ini input boolean; R3Lt_Step2_ini input boolean; R3Lt_Step1_done input boolean; R3Lt_Step2_done input boolean; R3Lt_Step1En output boolean; R3Lt_Step2En output boolean
